simulink model "AUV_APF"  (R2020b)
settings: Solver=VariableStepAuto  StartTime=0.0  StopTime=400  FixedStep=0.1  MaxStep=0.5  RelTol=1e-3
libraries: pid_lib x4
settings Model: Creator=shanerutherford  LastModifiedBy=shanerutherford
settings SolverCC: ZeroCrossAlgorithm=Adaptive
settings DebuggingCC: MaskedZcDiagnostic=none  IgnoredZcDiagnostic=none

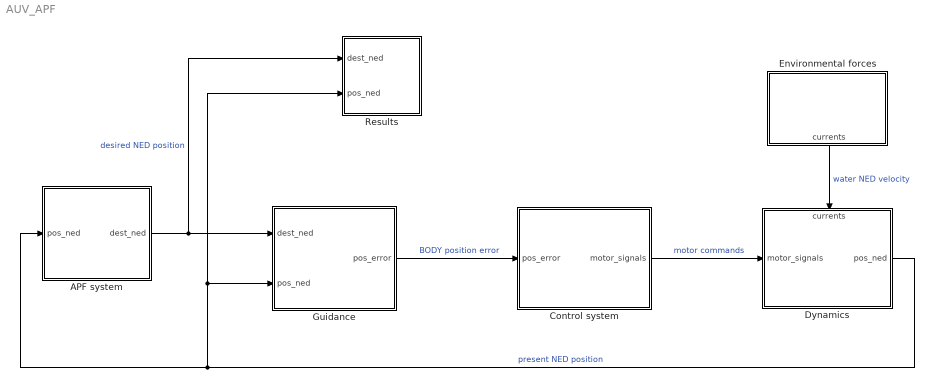
== system AUV_APF ==
  APF system : Subsystem
  Control system : Subsystem
  Dynamics : Subsystem
      settings: PortSchema="{\"entries\":[{\"content\":{\"sides\":[{\"content\":{\"connectorIds\":[\"In1\"]},\"type\":\"ConnectorPlacement.EquallySpacedRectSide\",\"uuid\":\"9ee444f3-b955-488d-8e49-640ea0f7df37\"},{\"content\":{\"connectorIds\":[\"Out1\"],\"side\":\"RIGHT\"},\"type\":\"ConnectorPlacement.EquallySpacedRectSide\",\"uuid\":\"ce4b5243-31e8-415d-aaa8-03cbb0c8065f\"},{\"content\":{\"connectorIds\":[\"In2\"],\"side\":\"TOP\"},\"type\":\"ConnectorPlacement.EquallySpacedRectSide\",\"uuid\":\"f69ed04b-67fd-4237-ab1a-d9f9564e83a0\"},{\"content\":{\"connectorIds\":[],\"side\":\"HIDDEN\"},\"type\":\"ConnectorPlacement.EquallySpacedRectSide\",\"uuid\":\"5b6b6d1e-b1c4-449c-9873-97d05fa29e3c\"}]},\"type\":\"ConnectorPlacement.EquallySpacedConnector\",\"uuid\":\"e4d51cd1-1a50-495c-8222-c38a5b01ba84\"}],\"packageUris\":[\"http://schema.mathworks.com/mf0/Connector/R2020b\"],\"version\":\"1.0\"}"
  Environmental forces : Subsystem
      settings: PortSchema="{\"entries\":[{\"content\":{\"sides\":[{\"content\":{\"connectorIds\":[]},\"type\":\"ConnectorPlacement.EquallySpacedRectSide\",\"uuid\":\"0dd98e89-aff4-433c-b28f-c29455b8a07d\"},{\"content\":{\"connectorIds\":[],\"side\":\"RIGHT\"},\"type\":\"ConnectorPlacement.EquallySpacedRectSide\",\"uuid\":\"953662a4-5b51-4456-b69c-eca28c97a39b\"},{\"content\":{\"connectorIds\":[],\"side\":\"TOP\"},\"type\":\"ConnectorPlacement.EquallySpacedRectSide\",\"uuid\":\"911274c2-620a-4054-9b06-c69233cda7b5\"},{\"content\":{\"connectorIds\":[\"Out1\"],\"side\":\"BOTTOM\"},\"type\":\"ConnectorPlacement.EquallySpacedRectSide\",\"uuid\":\"d1098ec8-c176-4eae-9d99-8b466f13cb7d\"},{\"content\":{\"connectorIds\":[],\"side\":\"HIDDEN\"},\"type\":\"ConnectorPlacement.EquallySpacedRectSide\",\"uuid\":\"331d0c74-f854-4ce9-a20e-6d7219b69b25\"}]},\"type\":\"ConnectorPlacement.EquallySpacedConnector\",\"uuid\":\"51f6c218-3b35-4d9f-b9df-5dfda31bafc0\"}],\"packageUris\":[\"http://schema.mathworks.com/mf0/Connector/R2020b\"],\"version\":\"1.0\"}"
  Guidance : Subsystem
  Results : Subsystem
  wires:
  Guidance/1(pos_error) -> Control system/1(pos_error)  "BODY position error"
  Dynamics/1(pos_ned) -> APF system/1(pos_ned), Guidance/2(pos_ned), Results/2(pos_ned)  "present NED position"
  Environmental forces/1(currents) -> Dynamics/2(currents)  "water NED velocity"
  Control system/1(motor_signals) -> Dynamics/1(motor_signals)  "motor commands"
  APF system/1(dest_ned) -> Guidance/1(dest_ned), Results/1(dest_ned)  "desired NED position"

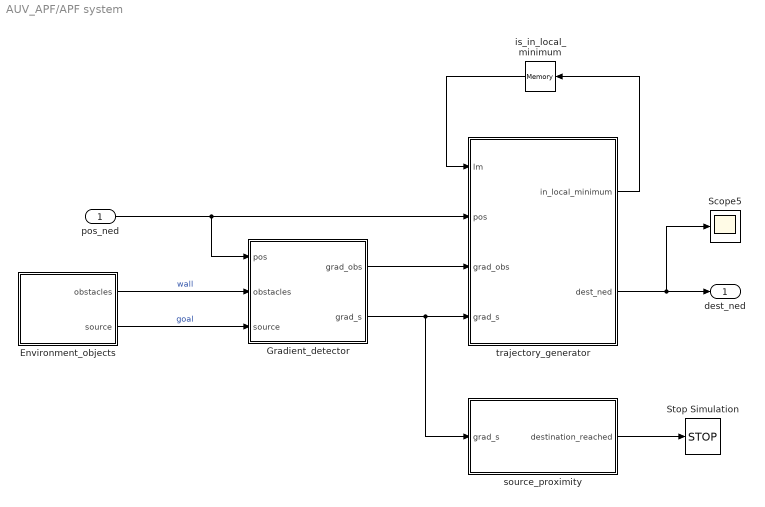
== system AUV_APF/APF system ==
  pos_ned : Inport
  Environment_objects : MATLAB Function  TreatAsAtomicUnit=on
  Gradient_detector : MATLAB Function  TreatAsAtomicUnit=on
  Scope5 : Scope
  Stop Simulation : Stop
  is_in_local_minimum : Memory
  source_proximity : MATLAB Function  TreatAsAtomicUnit=on
  trajectory_generator : MATLAB Function  TreatAsAtomicUnit=on
  dest_ned : Outport
  wires:
  trajectory_generator/1(in_local_minimum) -> is_in_local_minimum/1
  Environment_objects/2(source) -> Gradient_detector/3(source)  "goal"
  Environment_objects/1(obstacles) -> Gradient_detector/2(obstacles)  "wall"
  pos_ned/1 -> Gradient_detector/1(pos), trajectory_generator/2(pos)
  Gradient_detector/2(grad_s) -> trajectory_generator/4(grad_s), source_proximity/1(grad_s)
  Gradient_detector/1(grad_obs) -> trajectory_generator/3(grad_obs)
  trajectory_generator/2(dest_ned) -> Scope5/1, dest_ned/1
  source_proximity/1(destination_reached) -> Stop Simulation/1
  is_in_local_minimum/1 -> trajectory_generator/1(lm)

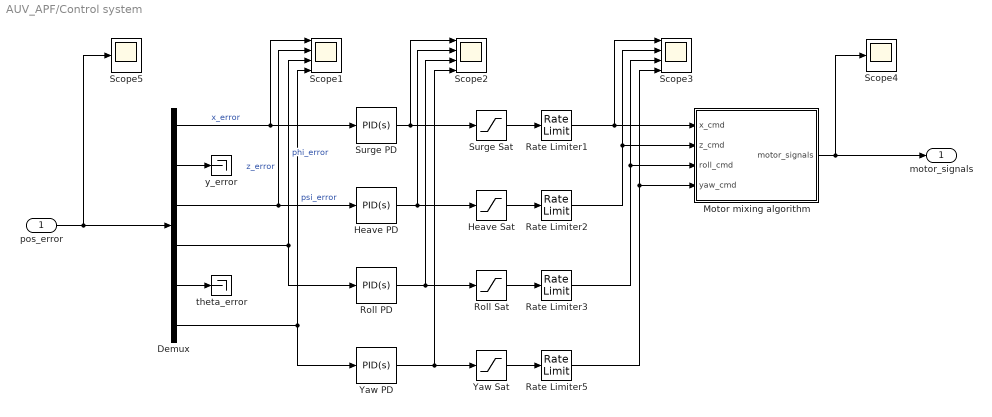
== system AUV_APF/Control system ==
  pos_error : Inport
  Demux : Demux  Outputs=6
  Heave PD : pid_lib/PID Controller  Controller=PID  Form=Parallel  TimeDomain=Continuous-time  UseExternalTs=off  SampleTime=-1  IntegratorMethod=Forward Euler  FilterMethod=Forward Euler  ControllerParametersSource=internal  P=10  I=0  D=5  UseFilter=on  N=100  TunerSelectOption=Transfer Function Based (PID Tuner App)  InitialConditionSource=internal  InitialConditionForIntegrator=0  InitialConditionForFilter=0  DifferentiatorICPrevScaledInput=0  ExternalReset=none  TrackingMode=off  Kt=1  LimitOutput=on  SatLimitsSource=internal  UpperSaturationLimit=100  LowerSaturationLimit=-100  LinearizeAsGain=on  AntiWindupMode=none  Kb=1  POutMin=[]  POutMax=[]  IOutMin=[]  IOutMax=[]  DOutMin=[]  DOutMax=[]  NOutMin=[]  NOutMax=[]  SumOutMin=[]  SumOutMax=[]  SaturationOutMin=[]  SaturationOutMax=[]  PParamMin=[]  PParamMax=[]  IParamMin=[]  IParamMax=[]  DParamMin=[]  DParamMax=[]  NParamMin=[]  NParamMax=[]  KbParamMin=[]  KbParamMax=[]  KtParamMin=[]  KtParamMax=[]  KbOutMin=[]  KbOutMax=[]  KtOutMin=[]  KtOutMax=[]  IntegratorOutMin=[]  IntegratorOutMax=[]  FilterOutMin=[]  FilterOutMax=[]  SumI1OutMin=[]  SumI1OutMax=[]  SumI2OutMin=[]  SumI2OutMax=[]  SumI3OutMin=[]  SumI3OutMax=[]  SumI4OutMin=[]  SumI4OutMax=[]  SumDOutMin=[]  SumDOutMax=[]  DifferentiatorOutMin=[]  DifferentiatorOutMax=[]  FilterDiffOutCoefMin=[]  FilterDiffOutCoefMax=[]  ReciprocalOutMin=[]  ReciprocalOutMax=[]  SumDenOutMin=[]  SumDenOutMax=[]  SumNumOutMin=[]  SumNumOutMax=[]  DivideOutMin=[]  DivideOutMax=[]  UdiffTsProdOutMin=[]  UdiffTsProdOutMax=[]  NTsProdOutMin=[]  NTsProdOutMax=[]  UintegralTsProdOutMin=[]  UintegralTsProdOutMax=[]  UngainTsProdOutMin=[]  UngainTsProdOutMax=[]  IntegratorContinuousStateAttributes=''  IntegratorStateMustResolveToSignalObject=off  IntegratorRTWStateStorageClass=Auto  FilterContinuousStateAttributes=''  FilterStateMustResolveToSignalObject=off  FilterRTWStateStorageClass=Auto  ParallelPVariant=InternalParameters  IdealPVariant=Disabled  IVariant=InternalParameters  DVariant=InternalParameters  IntegratorVariant=Continuous  SatVariant=Enabled  AWVariant=Passthrough  PCopyVariant=Disabled  TRVariant=Disabled  FdbkBlocksVariant=Forward  IdealPFdbkVariant=Disabled  SatFdbkVariant=Disabled  DerivativeFilterVariant=ContFilter  NVariant=InternalParameters  NCopyVariant=Disabled  FilterICVariant=InternalICsFilter  IntegratorICVariant=InternalICs  ExternalResetVariant=Disabled  TRSumVariant=Passthrough  SumFdbkVariant=Disabled  SumVariant=Sum_PID  TsampFilterVariant=InternalTs  TsampNgainVariant=Passthrough  TsampIntegralVariant=Passthrough  ExternalSaturationOutDataTypeStr=Inherit: Same as second input
  Heave Sat : Saturate  UpperLimit=40  LowerLimit=-40  ZeroCross=off
  Motor mixing algorithm : MATLAB Function  TreatAsAtomicUnit=on
  Rate Limiter{1..3,5} (4 alike) : RateLimiter  RisingSlewLimit=20  FallingSlewLimit=-20  SampleTimeMode=inherited
  Roll PD : pid_lib/PID Controller  Controller=PID  Form=Parallel  TimeDomain=Continuous-time  UseExternalTs=off  SampleTime=-1  IntegratorMethod=Forward Euler  FilterMethod=Forward Euler  ControllerParametersSource=internal  P=20  I=0  D=10  UseFilter=on  N=100  TunerSelectOption=Transfer Function Based (PID Tuner App)  InitialConditionSource=internal  InitialConditionForIntegrator=0  InitialConditionForFilter=0  DifferentiatorICPrevScaledInput=0  ExternalReset=none  TrackingMode=off  Kt=1  LimitOutput=on  SatLimitsSource=internal  UpperSaturationLimit=100  LowerSaturationLimit=-100  LinearizeAsGain=on  AntiWindupMode=none  Kb=1  POutMin=[]  POutMax=[]  IOutMin=[]  IOutMax=[]  DOutMin=[]  DOutMax=[]  NOutMin=[]  NOutMax=[]  SumOutMin=[]  SumOutMax=[]  SaturationOutMin=[]  SaturationOutMax=[]  PParamMin=[]  PParamMax=[]  IParamMin=[]  IParamMax=[]  DParamMin=[]  DParamMax=[]  NParamMin=[]  NParamMax=[]  KbParamMin=[]  KbParamMax=[]  KtParamMin=[]  KtParamMax=[]  KbOutMin=[]  KbOutMax=[]  KtOutMin=[]  KtOutMax=[]  IntegratorOutMin=[]  IntegratorOutMax=[]  FilterOutMin=[]  FilterOutMax=[]  SumI1OutMin=[]  SumI1OutMax=[]  SumI2OutMin=[]  SumI2OutMax=[]  SumI3OutMin=[]  SumI3OutMax=[]  SumI4OutMin=[]  SumI4OutMax=[]  SumDOutMin=[]  SumDOutMax=[]  DifferentiatorOutMin=[]  DifferentiatorOutMax=[]  FilterDiffOutCoefMin=[]  FilterDiffOutCoefMax=[]  ReciprocalOutMin=[]  ReciprocalOutMax=[]  SumDenOutMin=[]  SumDenOutMax=[]  SumNumOutMin=[]  SumNumOutMax=[]  DivideOutMin=[]  DivideOutMax=[]  UdiffTsProdOutMin=[]  UdiffTsProdOutMax=[]  NTsProdOutMin=[]  NTsProdOutMax=[]  UintegralTsProdOutMin=[]  UintegralTsProdOutMax=[]  UngainTsProdOutMin=[]  UngainTsProdOutMax=[]  IntegratorContinuousStateAttributes=''  IntegratorStateMustResolveToSignalObject=off  IntegratorRTWStateStorageClass=Auto  FilterContinuousStateAttributes=''  FilterStateMustResolveToSignalObject=off  FilterRTWStateStorageClass=Auto  ParallelPVariant=InternalParameters  IdealPVariant=Disabled  IVariant=InternalParameters  DVariant=InternalParameters  IntegratorVariant=Continuous  SatVariant=Enabled  AWVariant=Passthrough  PCopyVariant=Disabled  TRVariant=Disabled  FdbkBlocksVariant=Forward  IdealPFdbkVariant=Disabled  SatFdbkVariant=Disabled  DerivativeFilterVariant=ContFilter  NVariant=InternalParameters  NCopyVariant=Disabled  FilterICVariant=InternalICsFilter  IntegratorICVariant=InternalICs  ExternalResetVariant=Disabled  TRSumVariant=Passthrough  SumFdbkVariant=Disabled  SumVariant=Sum_PID  TsampFilterVariant=InternalTs  TsampNgainVariant=Passthrough  TsampIntegralVariant=Passthrough  ExternalSaturationOutDataTypeStr=Inherit: Same as second input
  Roll Sat : Saturate  UpperLimit=40  LowerLimit=-40  ZeroCross=off
  Scope1 : Scope  NumInputPorts=4
  Scope2 : Scope  NumInputPorts=4
  Scope3 : Scope  NumInputPorts=4
  Scope4 : Scope
  Scope5 : Scope
  Surge PD : pid_lib/PID Controller  Controller=PID  Form=Parallel  TimeDomain=Continuous-time  UseExternalTs=off  SampleTime=-1  IntegratorMethod=Forward Euler  FilterMethod=Forward Euler  ControllerParametersSource=internal  P=10  I=0  D=5  UseFilter=on  N=100  TunerSelectOption=Transfer Function Based (PID Tuner App)  InitialConditionSource=internal  InitialConditionForIntegrator=0  InitialConditionForFilter=0  DifferentiatorICPrevScaledInput=0  ExternalReset=none  TrackingMode=off  Kt=1  LimitOutput=on  SatLimitsSource=internal  UpperSaturationLimit=100  LowerSaturationLimit=-100  LinearizeAsGain=on  AntiWindupMode=none  Kb=1  POutMin=[]  POutMax=[]  IOutMin=[]  IOutMax=[]  DOutMin=[]  DOutMax=[]  NOutMin=[]  NOutMax=[]  SumOutMin=[]  SumOutMax=[]  SaturationOutMin=[]  SaturationOutMax=[]  PParamMin=[]  PParamMax=[]  IParamMin=[]  IParamMax=[]  DParamMin=[]  DParamMax=[]  NParamMin=[]  NParamMax=[]  KbParamMin=[]  KbParamMax=[]  KtParamMin=[]  KtParamMax=[]  KbOutMin=[]  KbOutMax=[]  KtOutMin=[]  KtOutMax=[]  IntegratorOutMin=[]  IntegratorOutMax=[]  FilterOutMin=[]  FilterOutMax=[]  SumI1OutMin=[]  SumI1OutMax=[]  SumI2OutMin=[]  SumI2OutMax=[]  SumI3OutMin=[]  SumI3OutMax=[]  SumI4OutMin=[]  SumI4OutMax=[]  SumDOutMin=[]  SumDOutMax=[]  DifferentiatorOutMin=[]  DifferentiatorOutMax=[]  FilterDiffOutCoefMin=[]  FilterDiffOutCoefMax=[]  ReciprocalOutMin=[]  ReciprocalOutMax=[]  SumDenOutMin=[]  SumDenOutMax=[]  SumNumOutMin=[]  SumNumOutMax=[]  DivideOutMin=[]  DivideOutMax=[]  UdiffTsProdOutMin=[]  UdiffTsProdOutMax=[]  NTsProdOutMin=[]  NTsProdOutMax=[]  UintegralTsProdOutMin=[]  UintegralTsProdOutMax=[]  UngainTsProdOutMin=[]  UngainTsProdOutMax=[]  IntegratorContinuousStateAttributes=''  IntegratorStateMustResolveToSignalObject=off  IntegratorRTWStateStorageClass=Auto  FilterContinuousStateAttributes=''  FilterStateMustResolveToSignalObject=off  FilterRTWStateStorageClass=Auto  ParallelPVariant=InternalParameters  IdealPVariant=Disabled  IVariant=InternalParameters  DVariant=InternalParameters  IntegratorVariant=Continuous  SatVariant=Enabled  AWVariant=Passthrough  PCopyVariant=Disabled  TRVariant=Disabled  FdbkBlocksVariant=Forward  IdealPFdbkVariant=Disabled  SatFdbkVariant=Disabled  DerivativeFilterVariant=ContFilter  NVariant=InternalParameters  NCopyVariant=Disabled  FilterICVariant=InternalICsFilter  IntegratorICVariant=InternalICs  ExternalResetVariant=Disabled  TRSumVariant=Passthrough  SumFdbkVariant=Disabled  SumVariant=Sum_PID  TsampFilterVariant=InternalTs  TsampNgainVariant=Passthrough  TsampIntegralVariant=Passthrough  ExternalSaturationOutDataTypeStr=Inherit: Same as second input
  Surge Sat : Saturate  UpperLimit=40  LowerLimit=-40  ZeroCross=off
  Yaw PD : pid_lib/PID Controller  Controller=PID  Form=Parallel  TimeDomain=Continuous-time  UseExternalTs=off  SampleTime=-1  IntegratorMethod=Forward Euler  FilterMethod=Forward Euler  ControllerParametersSource=internal  P=20  I=0  D=10  UseFilter=on  N=100  TunerSelectOption=Transfer Function Based (PID Tuner App)  InitialConditionSource=internal  InitialConditionForIntegrator=0  InitialConditionForFilter=0  DifferentiatorICPrevScaledInput=0  ExternalReset=none  TrackingMode=off  Kt=1  LimitOutput=on  SatLimitsSource=internal  UpperSaturationLimit=100  LowerSaturationLimit=-100  LinearizeAsGain=on  AntiWindupMode=none  Kb=1  POutMin=[]  POutMax=[]  IOutMin=[]  IOutMax=[]  DOutMin=[]  DOutMax=[]  NOutMin=[]  NOutMax=[]  SumOutMin=[]  SumOutMax=[]  SaturationOutMin=[]  SaturationOutMax=[]  PParamMin=[]  PParamMax=[]  IParamMin=[]  IParamMax=[]  DParamMin=[]  DParamMax=[]  NParamMin=[]  NParamMax=[]  KbParamMin=[]  KbParamMax=[]  KtParamMin=[]  KtParamMax=[]  KbOutMin=[]  KbOutMax=[]  KtOutMin=[]  KtOutMax=[]  IntegratorOutMin=[]  IntegratorOutMax=[]  FilterOutMin=[]  FilterOutMax=[]  SumI1OutMin=[]  SumI1OutMax=[]  SumI2OutMin=[]  SumI2OutMax=[]  SumI3OutMin=[]  SumI3OutMax=[]  SumI4OutMin=[]  SumI4OutMax=[]  SumDOutMin=[]  SumDOutMax=[]  DifferentiatorOutMin=[]  DifferentiatorOutMax=[]  FilterDiffOutCoefMin=[]  FilterDiffOutCoefMax=[]  ReciprocalOutMin=[]  ReciprocalOutMax=[]  SumDenOutMin=[]  SumDenOutMax=[]  SumNumOutMin=[]  SumNumOutMax=[]  DivideOutMin=[]  DivideOutMax=[]  UdiffTsProdOutMin=[]  UdiffTsProdOutMax=[]  NTsProdOutMin=[]  NTsProdOutMax=[]  UintegralTsProdOutMin=[]  UintegralTsProdOutMax=[]  UngainTsProdOutMin=[]  UngainTsProdOutMax=[]  IntegratorContinuousStateAttributes=''  IntegratorStateMustResolveToSignalObject=off  IntegratorRTWStateStorageClass=Auto  FilterContinuousStateAttributes=''  FilterStateMustResolveToSignalObject=off  FilterRTWStateStorageClass=Auto  ParallelPVariant=InternalParameters  IdealPVariant=Disabled  IVariant=InternalParameters  DVariant=InternalParameters  IntegratorVariant=Continuous  SatVariant=Enabled  AWVariant=Passthrough  PCopyVariant=Disabled  TRVariant=Disabled  FdbkBlocksVariant=Forward  IdealPFdbkVariant=Disabled  SatFdbkVariant=Disabled  DerivativeFilterVariant=ContFilter  NVariant=InternalParameters  NCopyVariant=Disabled  FilterICVariant=InternalICsFilter  IntegratorICVariant=InternalICs  ExternalResetVariant=Disabled  TRSumVariant=Passthrough  SumFdbkVariant=Disabled  SumVariant=Sum_PID  TsampFilterVariant=InternalTs  TsampNgainVariant=Passthrough  TsampIntegralVariant=Passthrough  ExternalSaturationOutDataTypeStr=Inherit: Same as second input
  Yaw Sat : Saturate  UpperLimit=40  LowerLimit=-40  ZeroCross=off
  theta_error : Terminator
  y_error : Terminator
  motor_signals : Outport
  wires:
  Demux/4 -> Scope1/3, Roll PD/1  "phi_error"
  Surge Sat/1 -> Rate Limiter1/1
  Demux/3 -> Scope1/2, Heave PD/1  "z_error"
  Roll Sat/1 -> Rate Limiter3/1
  Demux/6 -> Scope1/4, Yaw PD/1  "psi_error"
  Yaw Sat/1 -> Rate Limiter5/1
  Heave Sat/1 -> Rate Limiter2/1
  Demux/1 -> Scope1/1, Surge PD/1  "x_error"
  Demux/5 -> theta_error/1
  Demux/2 -> y_error/1
  Yaw PD/1 -> Scope2/4, Yaw Sat/1
  Roll PD/1 -> Roll Sat/1, Scope2/3
  Heave PD/1 -> Heave Sat/1, Scope2/2
  Surge PD/1 -> Surge Sat/1, Scope2/1
  Rate Limiter1/1 -> Scope3/1, Motor mixing algorithm/1(x_cmd)
  Rate Limiter2/1 -> Scope3/2, Motor mixing algorithm/2(z_cmd)
  Rate Limiter5/1 -> Motor mixing algorithm/4(yaw_cmd), Scope3/4
  Rate Limiter3/1 -> Scope3/3, Motor mixing algorithm/3(roll_cmd)
  Motor mixing algorithm/1(motor_signals) -> motor_signals/1, Scope4/1
  pos_error/1 -> Scope5/1, Demux/1

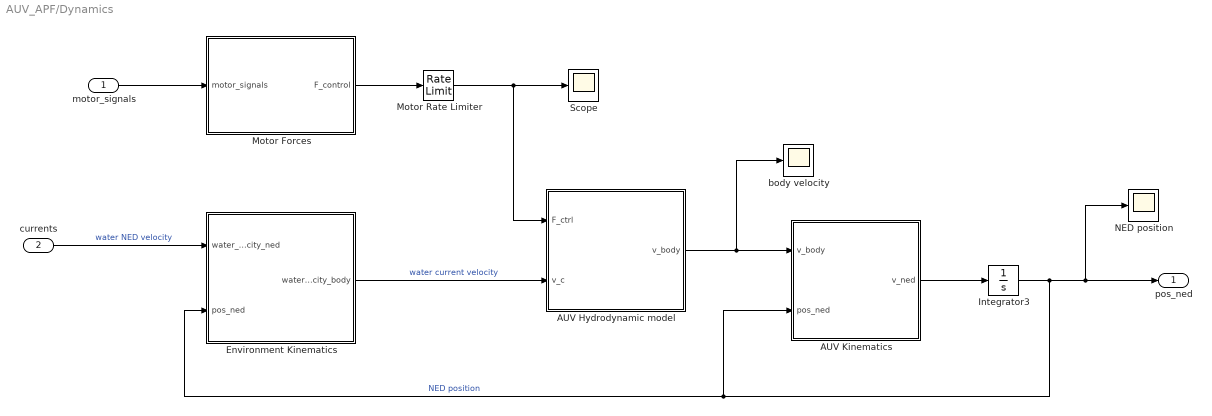
== system AUV_APF/Dynamics ==
  motor_signals : Inport
  currents : Inport  Port=2
  AUV Hydrodynamic model : Subsystem
  AUV Kinematics : MATLAB Function  TreatAsAtomicUnit=on
  Environment Kinematics : MATLAB Function  TreatAsAtomicUnit=on
  Integrator3 : Integrator
  Motor Forces : MATLAB Function  TreatAsAtomicUnit=on
  Motor Rate Limiter : RateLimiter  RisingSlewLimit=10  FallingSlewLimit=-10  SampleTimeMode=inherited
  NED position : Scope
  Scope : Scope
  body velocity : Scope
  pos_ned : Outport  PortDimensions=6
  wires:
  Integrator3/1 -> Environment Kinematics/2(pos_ned), AUV Kinematics/2(pos_ned), pos_ned/1, NED position/1  "NED position"
  Environment Kinematics/1(water_velocity_body) -> AUV Hydrodynamic model/2(v_c)  "water current velocity"
  AUV Kinematics/1(v_ned) -> Integrator3/1
  currents/1 -> Environment Kinematics/1(water_velocity_ned)  "water NED velocity"
  Motor Forces/1(F_control) -> Motor Rate Limiter/1
  motor_signals/1 -> Motor Forces/1(motor_signals)
  Motor Rate Limiter/1 -> AUV Hydrodynamic model/1(F_ctrl), Scope/1
  AUV Hydrodynamic model/1(v_body) -> body velocity/1, AUV Kinematics/1(v_body)

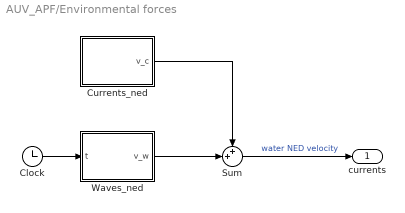
== system AUV_APF/Environmental forces ==
  Clock : Clock
  Currents_ned : MATLAB Function  TreatAsAtomicUnit=on
  Sum : Sum  Inputs=++|
  Waves_ned : MATLAB Function  TreatAsAtomicUnit=on
  currents : Outport
  wires:
  Sum/1 -> currents/1  "water NED velocity"
  Currents_ned/1(v_c) -> Sum/1
  Waves_ned/1(v_w) -> Sum/2
  Clock/1 -> Waves_ned/1(t)

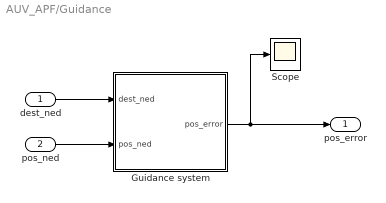
== system AUV_APF/Guidance ==
  dest_ned : Inport
  pos_ned : Inport  Port=2
  Guidance system : MATLAB Function  TreatAsAtomicUnit=on
  Scope : Scope
  pos_error : Outport
  wires:
  dest_ned/1 -> Guidance system/1(dest_ned)
  Guidance system/1(pos_error) -> pos_error/1, Scope/1
  pos_ned/1 -> Guidance system/2(pos_ned)

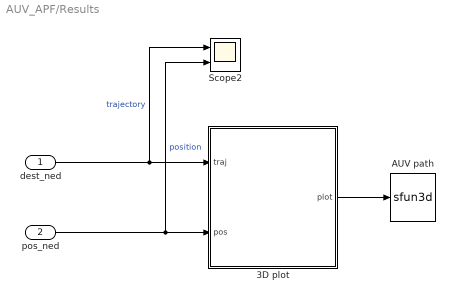
== system AUV_APF/Results ==
  dest_ned : Inport
  pos_ned : Inport  Port=2
  3D plot : MATLAB Function  TreatAsAtomicUnit=on
  AUV path : S-Function  LoadFcn=if exist('sfun3d','file'), sfun3d([],[],[],'LoadBlock'); end  FunctionName=sfun3d  Parameters=ax,T,np,cp,gd,ls,mk,mx,hd,tb  SFunctionDeploymentMode=off  EnableBusSupport=off  mask(3D Graph){np=2, ax=[-15 15 -15 15 -20 20], mx=1e4, T=-1, cp=[0, 0 15], gd=on, hd=on, tb=on, ls=-, mk=none}
      mask prompts: np "Number of moving points (lines)"; ax "Range: [xmin xmax  ymin ymax zmin zmax]"; mx "Max number of points in each line"; T "Sampling Time"; cp "Camera position (use [0 0 1] for 2D XY view)"; gd "Grid (on|off)"; hd "HeadMarkers (on|off)"; tb "Toolbar (on|off)"; ls "LineStyle"; mk "LineMarker"
      mask help:
      | This block plots the position of several points in the XYZ space. The input contains the coordinates of all the points (x1,y1,z1,x2,y2,z2,...).
      | The number of moving points (lines), the XYZ ranges, sampling time, camera position, and grid (among other things) can be set as mask parameters.
      settings: CopyFcn=if exist('sfun3d','file'), sfun3d([],[],[],'CopyBlock'); end  DeleteFcn=if exist('sfun3d','file'), sfun3d([],[],[],'DeleteBlock'); end  NameChangeFcn=if exist('sfun3d','file'), sfun3d([],[],[],'NameChange'); end
      mask Help:
      | This block plots the position of several points in the XYZ space. The input contains the coordinates of all the points (x1,y1,z1,x2,y2,z2,...).
      | The number of moving points (lines), the XYZ ranges, sampling time, camera position, and grid (among other things) can be set as mask parameters.
      mask TypeOptions ls: - | -- | : | -. | none
      mask TypeOptions mk: none | . | + | o | * | x | square | diamond | v | ^ | > | < | pentagram | hexagram
      mask Display: plot([.05 .95 .95 .05 .05],[.45 .45 .95 .95 .45], 0.5+cos(0:0.1:2*pi)*0.3,0.7+sin(0:0.1:2*pi)*0.2)
  Scope2 : Scope  NumInputPorts=2
  wires:
  3D plot/1(plot) -> AUV path/1
  pos_ned/1 -> Scope2/2, 3D plot/2(pos)  "position"
  dest_ned/1 -> Scope2/1, 3D plot/1(traj)  "trajectory"

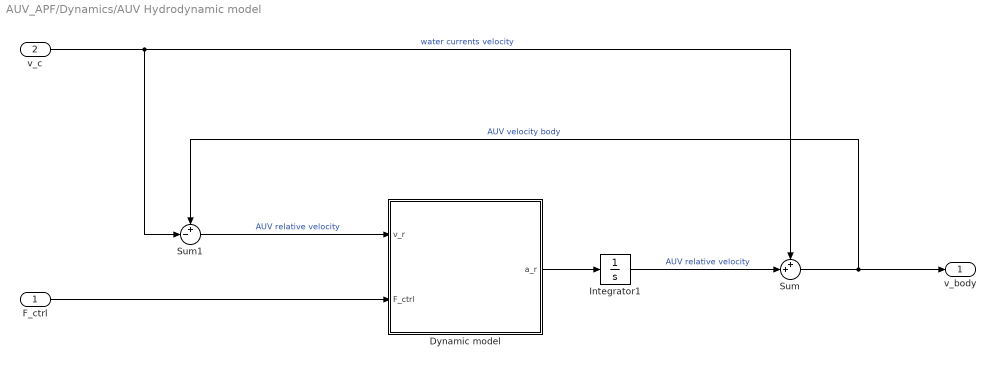
== system AUV_APF/Dynamics/AUV Hydrodynamic model ==
  F_ctrl : Inport
  v_c : Inport  Port=2
  Dynamic model : MATLAB Function  TreatAsAtomicUnit=on
  Integrator1 : Integrator
  Sum : Sum  Inputs=++|
  Sum1 : Sum  Inputs=+-|
  v_body : Outport
  wires:
  F_ctrl/1 -> Dynamic model/2(F_ctrl)
  Integrator1/1 -> Sum/2  "AUV relative velocity"
  v_c/1 -> Sum/1, Sum1/2  "water currents velocity"
  Dynamic model/1(a_r) -> Integrator1/1
  Sum1/1 -> Dynamic model/1(v_r)  "AUV relative velocity"
  Sum/1 -> Sum1/1, v_body/1  "AUV velocity body"

== matlab function AUV_APF/Control system/Motor mixing algorithm ==
  data: x_cmd input; motor_signals output size=[1, 4]; z_cmd input; roll_cmd input; yaw_cmd input
function motor_signals = fcn(x_cmd, z_cmd, roll_cmd, yaw_cmd)

% motor_limit is an arbitary value representing max signal level.
% This is scaled in the motor model so that a motor is at full power when
% its motor_signal is 40, and off when its motor_signal is 0.
motor_signal_max = 40; 

% Linear and rotational commands on one motor may combine to exceed the
% limit of that motor. In this situation, the rotational command is
% prioritised and the linear command is curtailed. 
if abs(x_cmd) + abs(yaw_cmd) > motor_signal_max
    x_cmd = sign(x_cmd) * (motor_signal_max - abs(yaw_cmd));
end
if abs(z_cmd) + abs(roll_cmd) > motor_signal_max
    z_cmd = sign(z_cmd) * (motor_signal_max - abs(roll_cmd));
end

front_right_motor = -z_cmd - roll_cmd;
front_left_motor = -z_cmd + roll_cmd;
back_right_motor = x_cmd - yaw_cmd;
back_left_motor = x_cmd + yaw_cmd;

motor_signals = [front_right_motor, front_left_motor, back_right_motor, back_left_motor];
end

== matlab function AUV_APF/APF system/trajectory_generator ==
  data: lm input; in_local_minimum output; pos input; grad_obs input; dest_ned output size=3; grad_s input
function [in_local_minimum, dest_ned]= fcn(lm, pos, grad_obs, grad_s)

    CONSIDER_OBSTACLES = 1;
    SPEED_SCALE = 0.8;        % scales AUV speed
   
    % Local minimum checks
    source_obs_angle_diff = atan2(norm(cross(grad_s, grad_obs)), dot(grad_s, grad_obs)); % Angle between gradients
    obs_angle_diff = atan2(norm(cross([0, 0, -1], grad_obs)), dot([0, 0, -1], grad_obs)); % Angle between wall and downwards axis
    
    in_local_minimum = lm;
    if in_local_minimum == 1
        % Check if AUV can exit wall following pattern
        if (norm(grad_obs) == 0) || (obs_angle_diff < 0.5)
           in_local_minimum = 0; 
        end
    else
        % Check if AUV is in a local minimum, and should enter a wall
        % following pattern
        MAG_LOW = 0.2;
        ANG_HIGH = 2.9;
        if (norm(grad_obs) > 0) && (source_obs_angle_diff > ANG_HIGH) && (obs_angle_diff > 1)
            in_local_minimum = 1;
        end
    end
    
    
    % Calculate an overall gradient
    if CONSIDER_OBSTACLES == 1
        if in_local_minimum == 1
            grad_obs_T = [grad_obs(2); -grad_obs(1); grad_obs(3)];
            gradient = cross(grad_obs, grad_obs_T);
        else
            
            a = atan2(norm(cross(grad_obs, grad_s)),dot(grad_obs, grad_s)); % Angle between gradients
            k = a/pi;           % scaling factor
            gradient =  k*grad_obs + (1-k)*grad_s;
%             gradient = grad_s + grad_obs;
        end
    else
        gradient = grad_s;
    end
    
    % Set new position
    if norm(gradient) < 0.001
        dest_ned = pos(1:3);
    else
        dest_ned = pos(1:3) + SPEED_SCALE * gradient / norm(gradient);
    end
end

== matlab function AUV_APF/Results/3D plot ==
  data: traj input; plot output; pos input
function plot = fcn(traj, pos)
 plot = [traj(2); traj(1); -traj(3); pos(2); pos(1); -pos(3)];

== matlab function AUV_APF/APF system/Gradient_detector ==
  data: grad_obs output; pos input; obstacles input; grad_s output; source input
function [grad_obs, grad_s] = fcn(pos, obstacles, source)

    % Calculate gradient due to obstacles
    % Find shortest distance between obstacle and position    
    if pos(1) < obstacles(1, 4) && pos(3) < obstacles(3, 4)
        % postion is to the bottom left of obstacle
        d_obs = obstacles(:, 4) - pos(1:3);

    elseif pos(1) < obstacles(1, 1) && pos(3) > obstacles(3, 1)
        % postion is to the top left of obstacle
        d_obs = obstacles(:, 1) - pos(1:3);

    elseif pos(1) > obstacles(1, 3) && pos(3) < obstacles(3, 3)
        % postion is to the bottom right of obstacle
        d_obs = obstacles(:, 3) - pos(1:3);

    elseif pos(1) > obstacles(1, 2) && pos(3) > obstacles(3, 2)
        % postion is to the top right of obstacle
        d_obs = obstacles(:, 2) - pos(1:3);

    elseif pos(1) < obstacles(1, 1)
        % postion is to the left of obstacle
        d_obs = [obstacles(1,1) - pos(1);
              obstacles(2,1) - pos(2);
              0];
    elseif pos(1) > obstacles(1, 2)
        % postion is to the right of obstacle
        d_obs = [obstacles(1, 2) - pos(1);
              obstacles(2, 2) - pos(2);
              0];
    elseif pos(3) < obstacles(3, 3)
        % postion is below obsticle
        d_obs = [0;
              obstacles(2, 3) - pos(2);
              obstacles(3, 3) - pos(3)];
    elseif pos(3) > obstacles(3, 2)
        % postion is above obstacle
        d_obs = [0;
              obstacles(2, 2) - pos(2);
              obstacles(3, 2) - pos(3)];
    else
        % position overlaps on y axis
        d_obs = [0;
              obstacles(2, 1) - pos(2);
              0];
    end
    
    s_max = 2;  % Scaling factor to override source
    Limit = 5;    % Set values to zero beyond this range
    
    if norm(d_obs) < Limit
        grad_obs = -s_max/(1+norm(d_obs)) * d_obs/norm(d_obs);
    else
        grad_obs = [0;0;0];
    end

    
    % Calculate gradient due to source
    s_source = 10;
    d_source = source - pos(1:3);

    grad_s = (1 - s_source/(s_source+norm(d_source))) * d_source/norm(d_source);

== matlab function AUV_APF/Environmental forces/Currents_ned ==
  data: v_c output
function v_c = fcn()
    % currents are irrotational
    % v_c is the ned velocity of the current     

%     v_c = [1; 0; 0];
    v_c = [0; 0; 0];
end

== matlab function AUV_APF/Dynamics/Motor Forces ==
  data: F_control output size=6; motor_signals input
function F_control = fcn(motor_signals)
% x, y, and z axis relates to local front, starboard, and down directions
% phi, theta, and psi represents roll, pitch, and yaw 

% assuming that the force produced by each motor is proportonal to the
% signal voltage

motor_signal_max = 40;
motor_thrust_max = 1.36;    % (N) See Propulsion_forces.m for estimate

k = motor_thrust_max/motor_signal_max;

FrontRight_m = k*motor_signals(1);
FrontLeft_m = k*motor_signals(2);
BackRight_m = k*motor_signals(3);
BackLeft_m = k*motor_signals(4);

F_control = [
    BackRight_m+BackLeft_m; 
    0;                          % AUV cannot move in y direction
    -FrontRight_m-FrontLeft_m;  % positive z is downward 
    FrontLeft_m-FrontRight_m;   % positive rotation is clockwise
    0;                      	% AUV cannot pitch 
    BackLeft_m-BackRight_m;
];

== matlab function AUV_APF/Dynamics/AUV Kinematics ==
  data: v_body input; pos_ned input; v_ned output
function v_ned = fcn(v_body, pos_ned)
% Transform from AUV body frame to NED frame

    J = Jacobian(pos_ned(4), pos_ned(5), pos_ned(6)); 
    v_ned = J * v_body;
end

== matlab function AUV_APF/Environmental forces/Waves_ned ==
  data: v_w output; t input
function v_w = fcn(t)
    % currents are irrotational
    % v_w is the NED velocity of the water in the wave
    % sine function is used to generate the waves
    
    wave_period = 5; % time between each wave in seconds
    wave_amplitude = 0;
%     wave_amplitude = 0.1; % maximum water velocity of wave (m/s)
    
    wave_velocity = wave_amplitude * sin(t/(wave_period*pi));
    v_w = [0; 0; wave_velocity];
end

== matlab function AUV_APF/Guidance/Guidance system ==
  data: dest_ned input; pos_error output; pos_ned input
function pos_error = fcn(dest_ned, pos_ned)
    % note that x is north, y is east and z is down    
    N_error = dest_ned(1)-pos_ned(1);
    E_error = dest_ned(2)-pos_ned(2);
    D_error = dest_ned(3)-pos_ned(3);

    current_heading = pos_ned(6);
    desired_heading = atan2(E_error, N_error);

    % convert to body axis
    x_error = max([-1, N_error*cos(current_heading)+E_error*sin(current_heading)]);
    y_error = 0;
    z_error = D_error;

    roll_error = 0;
    pitch_error = 0;
    yaw_error = desired_heading - current_heading;
    
    while roll_error > pi
        roll_error = roll_error - 2*pi;
    end
    while roll_error < -pi
        roll_error = roll_error + 2*pi;
    end

    while yaw_error > pi
        yaw_error = yaw_error - 2*pi;
    end
    while yaw_error < -pi
        yaw_error = yaw_error + 2*pi;
    end
    
    % Scale x_error down when yaw_error is high 
    k_angle = yaw_error*3;
    if k_angle > pi || k_angle < -pi
        k_angle = pi;
    end
     
    k = 0.5*cos(k_angle)+0.5;
    x_error = x_error*k;
        
    pos_error = [x_error; y_error; z_error; roll_error; pitch_error; yaw_error];
end

== matlab function AUV_APF/APF system/Environment_objects ==
  data: obstacles output; source output
function [obstacles, source] = fcn()

% Source that detector is looking for
% source = [5; 20; 10];
source = [10; 50; 30];

% obstacle to be avoided 
% coordinates ordered in top-left, top-right, bottom-right,  bottom-left
% obstacles = [
%      -1, 4, 4, -1; 
%      -5, -5, -5, -5; 
%      11, 11, 3, 3
% ];
obstacles = [
     -5, 15, 15, -5; 
     20, 20, 20, 20; 
     15, 15, 5, 5
];

== matlab function AUV_APF/Dynamics/Environment Kinematics ==
  data: water_velocity_ned input; pos_ned input; water_velocity_body output size=6
function water_velocity_body = fcn(water_velocity_ned, pos_ned)
    R = rotateZYX(pos_ned(4), pos_ned(5), pos_ned(6));
    w_v =  R \ water_velocity_ned;
    water_velocity_body = [w_v(1); w_v(2); w_v(3); 0; 0; 0];
end

== matlab function AUV_APF/APF system/source_proximity ==
  data: grad_s input; destination_reached output
function destination_reached = fcn(grad_s)

    % End simulation if source is very close
    destination_reached = 0;
    arrival_term = 1 - norm(grad_s);
    if arrival_term > 0.95
        destination_reached = 1;
    end

== matlab function AUV_APF/Dynamics/AUV Hydrodynamic model/Dynamic model ==
  data: v_r input; F_ctrl input; a_r output size=6
function a_r = fcn(v_r, F_ctrl)
% v_r is velocity of the AUV relative to the water
% Uses AUV dynamic model file to get acceleration of the AUV relative to
% the water

% Uncomment to view simulaiton with wave only forces
% F_ctrl(1) = 0;
% F_ctrl(2) = 0;
% F_ctrl(3) = 0;

[M, C, D, g] = AUV_dynamic_model(v_r);    
a_r = M\(F_ctrl - C*v_r - D*v_r - g);
